simulink model "lorentzsimu_control"  (R2017b)
settings: Solver=ode4  StartTime=0.0  StopTime=15  FixedStep=1e-5  RelTol=1e-3
values from neighbouring files (symbols this model uses):
  beta = 2    [TEA_Ejercicios0_control_barco_sMatlab.m]    (also in lorentz.m = 2.66666666667; lorentzlqr.m = 2.66666666667)
  init = Pnumerico(1,:)+1    [lorentzlqr.m]
  KCC = place(A1,B1,[-13.85, -0.8 + 0.816*1i, -0.8 - 0.816*1i])    [lorentzlqr.m]
  KClqr = lqr(A1,B1,Qc,Rc)    [lorentzlqr.m]
  Pnumerico = double(Psimbolico)    [lorentzlqr.m]
  rho = 28    [lorentz.m]    (also in lorentzlqr.m)
  sat = 5    [lorentzlqr.m]
  sigma = 10    [lorentz.m]    (also in lorentzlqr.m)
  tau_act = 0.01    [lorentzlqr.m]
settings Model: Creator=pablo  LastModifiedBy=pablo

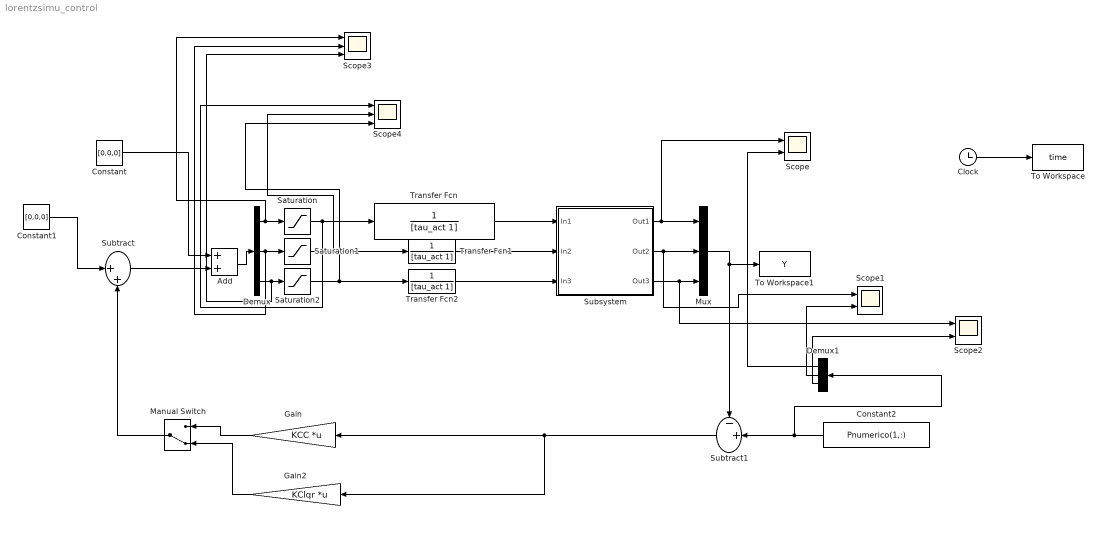
== system lorentzsimu_control ==
  Add : Sum
  Clock : Clock
  Constant : Constant  Value=[0,0,0]
  Constant1 : Constant  Value=[0,0,0]
  Constant2 : Constant  Value=Pnumerico(1,:)
  Demux : Demux  Outputs=3
  Demux1 : Demux  Outputs=3
  Gain : Gain  Gain=KCC  Multiplication=Matrix(K*u) (u vector)
  Gain2 : Gain  Gain=KClqr  Multiplication=Matrix(K*u) (u vector)
  Manual Switch : ManualSwitch  CurrentSetting=0
  Mux : Mux  Inputs=3
  Saturation : Saturate  UpperLimit=sat  LowerLimit=-sat
  Saturation1 : Saturate  UpperLimit=sat  LowerLimit=-sat
  Saturation2 : Saturate  UpperLimit=sat  LowerLimit=-sat
  Scope : Scope  NumInputPorts=2
  Scope1 : Scope  NumInputPorts=2
  Scope2 : Scope  NumInputPorts=2
  Scope3 : Scope  NumInputPorts=3
  Scope4 : Scope  NumInputPorts=3
  Subsystem : Subsystem
  Subtract : Sum  Inputs=|++
  Subtract1 : Sum  Inputs=-+|
  To Workspace : ToWorkspace  VariableName=time  SaveFormat=Timeseries  SampleTime=-1
  To Workspace1 : ToWorkspace  VariableName=Y  SaveFormat=Timeseries  SampleTime=-1
  Transfer Fcn : TransferFcn  Denominator=[tau_act 1]
  Transfer Fcn1 : TransferFcn  Denominator=[tau_act 1]
  Transfer Fcn2 : TransferFcn  Denominator=[tau_act 1]
  wires:
  Clock/1 -> To Workspace/1
  Demux/1 -> Saturation/1, Scope3/1
  Demux/2 -> Saturation1/1, Scope3/2
  Demux/3 -> Saturation2/1, Scope3/3
  Add/1 -> Demux/1
  Subsystem/1(Out1) -> Scope/1, Mux/1
  Subsystem/2(Out2) -> Scope1/1, Mux/2
  Subsystem/3(Out3) -> Scope2/1, Mux/3
  Mux/1 -> Subtract1/1, To Workspace1/1
  Subtract/1 -> Add/2
  Constant2/1 -> Subtract1/2, Demux1/1
  Constant/1 -> Add/1
  Constant1/1 -> Subtract/1
  Demux1/1 -> Scope/2
  Demux1/2 -> Scope1/2
  Demux1/3 -> Scope2/2
  Saturation/1 -> Transfer Fcn/1, Scope4/1
  Saturation1/1 -> Transfer Fcn1/1, Scope4/2
  Saturation2/1 -> Transfer Fcn2/1, Scope4/3
  Transfer Fcn/1 -> Subsystem/1(In1)
  Transfer Fcn1/1 -> Subsystem/2(In2)
  Transfer Fcn2/1 -> Subsystem/3(In3)
  Subtract1/1 -> Gain/1, Gain2/1
  Gain2/1 -> Manual Switch/2
  Manual Switch/1 -> Subtract/2
  Gain/1 -> Manual Switch/1

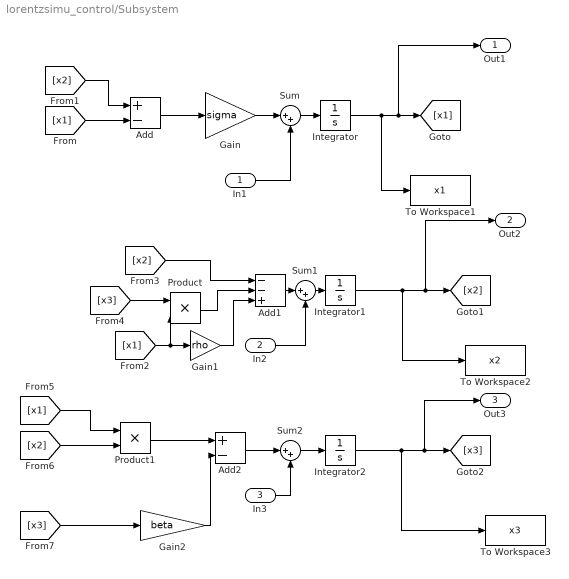
== system lorentzsimu_control/Subsystem ==
  In1 : Inport
  In2 : Inport  Port=2
  In3 : Inport  Port=3
  Add : Sum  Inputs=+-
  Add1 : Sum  Inputs=--+
  Add2 : Sum  Inputs=+-
  Gain : Gain  Gain=sigma
  Gain1 : Gain  Gain=rho
  Gain2 : Gain  Gain=beta
  Integrator : Integrator  InitialCondition=init(1)
  Integrator1 : Integrator  InitialCondition=init(2)
  Integrator2 : Integrator  InitialCondition=init(3)
  Product : Product
  Product1 : Product
  Sum : Sum  Inputs=|++
  Sum1 : Sum  Inputs=|++
  Sum2 : Sum  Inputs=|++
  To Workspace1 : ToWorkspace  VariableName=x1  SampleTime=-1
  To Workspace2 : ToWorkspace  VariableName=x2  SampleTime=-1
  To Workspace3 : ToWorkspace  VariableName=x3  SampleTime=-1
  Out1 : Outport
  Out2 : Outport  Port=2
  Out3 : Outport  Port=3
  wires:
  [x1] -> Product/2, Gain1/1
  Integrator/1 -> To Workspace1/1, Out1/1, [x1]
  [x2] -> Add/1
  [x1] -> Add/2
  Add/1 -> Gain/1
  Gain1/1 -> Add1/3
  [x2] -> Add1/1
  Product/1 -> Add1/2
  [x3] -> Product/1
  Integrator1/1 -> To Workspace2/1, Out2/1, [x2]
  Product1/1 -> Add2/1
  [x1] -> Product1/1
  [x2] -> Product1/2
  [x3] -> Gain2/1
  Gain2/1 -> Add2/2
  Integrator2/1 -> To Workspace3/1, Out3/1, [x3]
  Gain/1 -> Sum/1
  Sum/1 -> Integrator/1
  In1/1 -> Sum/2
  Add1/1 -> Sum1/1
  Sum1/1 -> Integrator1/1
  In2/1 -> Sum1/2
  In3/1 -> Sum2/2
  Add2/1 -> Sum2/1
  Sum2/1 -> Integrator2/1
